simulink model "MassSpringDamper"  (R2021a)
settings: Solver=FixedStepAuto  StartTime=0.0  StopTime=10.0  FixedStep=0.01  RelTol=1e-3
model workspace (MAT data in the model file):
  b = 1
  k = 1
  m = 1
libraries: fl_lib x9, nesl_utility x6, sm_lib x4, fl_ps_legacy_lib x1
settings Model: Creator=yleong  LastModifiedBy=smuckati
settings SolverCC: AlgebraicLoopSolver=TrustRegion
settings OptimizationCC: DefaultParameterBehavior=Inlined  UseDivisionForNetSlopeComputation=on  EnhancedBackFolding=on  PassReuseOutputArgsAs=Individual arguments  OptimizeBlockOrder=speed  DifferentSizesBufferReuse=on  OptimizationCustomize=off  EfficientTunableParamExpr=on
settings DebuggingCC: ParameterTunabilityLossMsg=error  SFMachineParentedDataDiag=warning  ArithmeticOperatorsInVariantConditions=warning
settings SFSimCC: MATLABDynamicMemAlloc=off  CustomCodeUndefinedFunction=UseInterfaceOnly
settings RTWCC: SystemTargetFile=ert.tlc  TemplateMakefile=ert_default_tmf  IncludeHyperlinkInReport=on  CodeExecutionProfiling=on  CodeProfilingSaveOptions=AllData
settings CodeAppCC: ForceParamTrailComments=on  IgnoreCustomStorageClasses=off  OperatorAnnotations=on  SimulinkDataObjDesc=on  SFDataObjDesc=on  InsertBlockDesc=on
settings ERTTargetCC: TargetLangStandard=C99 (ISO)  GenerateSampleERTMain=on  InlinedParameterPlacement=NonHierarchical  ERTCustomFileTemplate=example_file_process.tlc

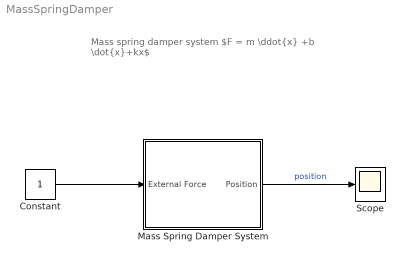
== system MassSpringDamper ==
  note: Mass spring damper system
      |
      | $F = m \ddot{x} +b \dot{x}+kx$
  " Scope " : Scope
  Constant : Constant
  Mass Spring Damper System : Subsystem  Variant=on  VariantControlMode=label  LabelModeActiveChoice=Equation of motion
  wires:
  Mass Spring Damper System/1(Position) -> " Scope "/1  "position"
  Constant/1 -> Mass Spring Damper System/1(" External Force")

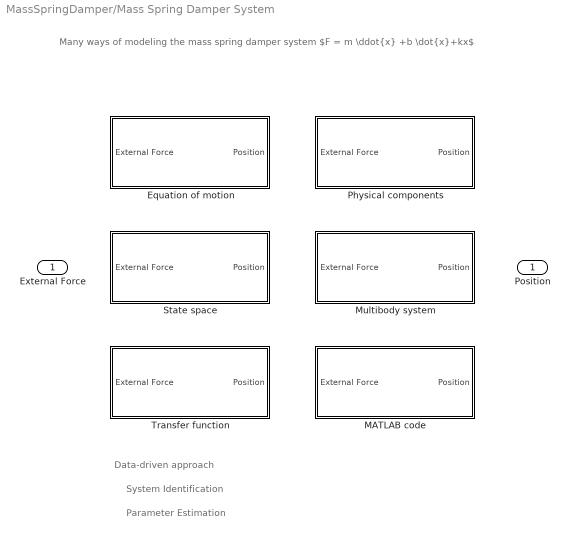
== system MassSpringDamper/Mass Spring Damper System ==
  note: Parameter Estimation
  note: Data-driven approach
  note: System Identification
  note: Many ways of modeling the mass spring damper system
      |
      | $F = m \ddot{x} +b \dot{x}+kx$
  " External Force" : Inport
  Equation of motion : Subsystem  VariantControl=Equation of motion
  MATLAB code : Subsystem  VariantControl=MATLAB code
  Multibody system : Subsystem  VariantControl=Multibody system
  Physical components : Subsystem  VariantControl=Physical components
  State space : Subsystem  VariantControl=State space
  Transfer function : Subsystem  VariantControl=Transfer function
  Position : Outport  VectorParamsAs1DForOutWhenUnconnected=off

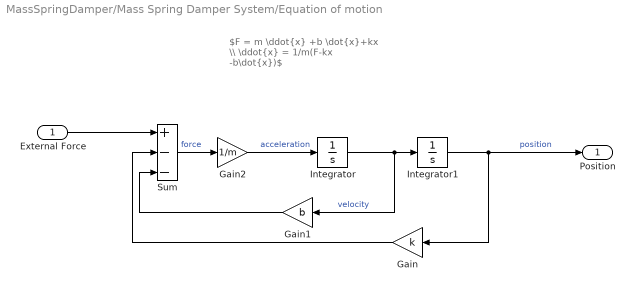
== system MassSpringDamper/Mass Spring Damper System/Equation of motion ==
  note: $F = m \ddot{x} +b \dot{x}+kx \\ \ddot{x} = 1/m(F-kx -b\dot{x})$
  " External Force" : Inport
  Gain : Gain  Gain=k
  Gain1 : Gain  Gain=b
  Gain2 : Gain  Gain=1/m
  Integrator : Integrator
  Integrator1 : Integrator
  Sum : Sum  Inputs=+--
  Position : Outport  VectorParamsAs1DForOutWhenUnconnected=off
  wires:
  Sum/1 -> Gain2/1  "force"
  Integrator1/1 -> Position/1, Gain/1  "position"
  Gain1/1 -> Sum/3
  Integrator/1 -> Gain1/1, Integrator1/1  "velocity"
  Gain/1 -> Sum/2
  Gain2/1 -> Integrator/1  "acceleration"
  " External Force"/1 -> Sum/1

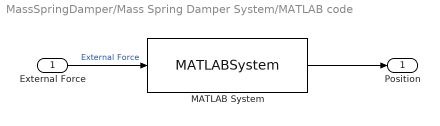
== system MassSpringDamper/Mass Spring Damper System/MATLAB code ==
  " External Force" : Inport
  MATLAB System : MATLABSystem  System=MassSpringDamperSystem  m=1  k=0.1  b=0.1  SimulateUsing=Code generation
      mask Type: MassSpringDamperSystem
      mask Display:
      | disp('MassSpringDamperSystem');
      | port_label('input',1,'u');
      | port_label('output',1,'y');
  Position : Outport  VectorParamsAs1DForOutWhenUnconnected=off
  wires:
  " External Force"/1 -> MATLAB System/1  "External Force"
  MATLAB System/1 -> Position/1

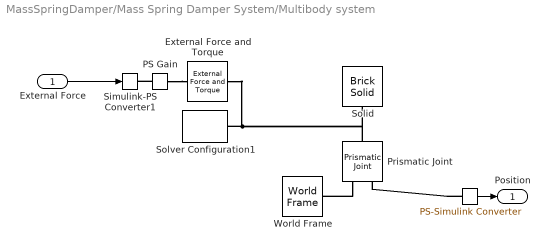
== system MassSpringDamper/Mass Spring Damper System/Multibody system ==
  " External Force" : Inport
  " " : nesl_utility/PS-Simulink Converter  PhysicalDomain=network_engine_domain  SubClassName=ps_output  LeftPortType=input  RightPortType=output  PseudoPeriodic=off  Frequencies=[]  Unit=1  AffineConversion=off
      settings: SourceProductBaseCode=PW,SS
  External Force and Torque : sm_lib/Forces and Torques/External Force and Torque  ForceResolutionFrame=AttachedFrame  EnableForceX=off  EnableForceY=off  EnableForceZ=on  EnableForce=off  TorqueResolutionFrame=AttachedFrame  EnableTorqueX=off  EnableTorqueY=off  EnableTorqueZ=off  EnableTorque=off
  PS Gain : fl_ps_legacy_lib/Legacy Physical Signals/Functions/PS Gain  gain=-1
  Prismatic Joint : sm_lib/Joints/Prismatic Joint  JointMode=Normal  SenseConstraintForce=off  SenseConstraintForceX=off  SenseConstraintForceY=off  SenseConstraintForceZ=off  SenseConstraintTorque=off  SenseConstraintTorqueX=off  SenseConstraintTorqueY=off  SenseConstraintTorqueZ=off  SenseTotalForce=off  SenseTotalForceX=off  SenseTotalForceY=off  SenseTotalForceZ=off  SenseTotalTorque=off  SenseTotalTorqueX=off  SenseTotalTorqueY=off  SenseTotalTorqueZ=off  CompositeWrenchDir=FollowerOnBase  CompositeWrenchFrame=BaseFrame  EquilibriumPosition=0  EquilibriumPositionUnits=m  SpringStiffness=k  SpringStiffnessUnits=N/m  DampingCoefficient=b  DampingCoefficientUnits=N/(m/s)  TorqueActuationMode=NoTorque  MotionActuationMode=ComputedMotion  SensePosition=on  SenseVelocity=off  SenseAcceleration=off  SenseTorqueForce=off  SenseLowerLimitTorqueForce=off  SenseUpperLimitTorqueForce=off  LowerLimitSpecify=off  LowerLimitBound=-1  LowerLimitBoundUnits=m  LowerLimitStiffness=1e6  LowerLimitStiffnessUnits=N/m  LowerLimitDamping=1e3  LowerLimitDampingUnits=N/(m/s)  LowerLimitTransitionRegionWidth=1e-4  LowerLimitTransitionRegionWidthUnits=m  UpperLimitSpecify=off  UpperLimitBound=1  UpperLimitBoundUnits=m  UpperLimitStiffness=1e6  UpperLimitStiffnessUnits=N/m  UpperLimitDamping=1e3  UpperLimitDampingUnits=N/(m/s)  UpperLimitTransitionRegionWidth=1e-4  UpperLimitTransitionRegionWidthUnits=m  PositionTargetSpecify=off  PositionTargetPriority=High  PositionTargetValue=10  PositionTargetValueUnits=m  VelocityTargetSpecify=off  VelocityTargetPriority=High  VelocityTargetValue=0  VelocityTargetValueUnits=m/s
  Simulink-PS Converter1 : nesl_utility/Simulink-PS Converter  PhysicalDomain=network_engine_domain  SubClassName=ps_input  LeftPortType=input  RightPortType=output  PseudoPeriodic=off  Frequencies=[]  NoiseDistribution=none  NoiseParameters=[]  Unit=N  AffineConversion=off  FilteringAndDerivatives=provide  SimscapeFilterOrder=1  InputFilterTimeConstant=0.001  UdotUserProvided=0
      settings: SourceProductBaseCode=PW,SS
  Solid : sm_lib/Body Elements/Brick Solid  GraphicAmbientColor=[0.15 0.15 0.15 1.0]  BasedOnType=Mass  BrickDimensions=[1 1 1]  BrickDimensionUnits=m  CenterOfMass=[0 0 0]  CenterOfMassUnits=m  GraphicDiffuseColor=[0.5 0.5 0.5]  Density=1000  DensityUnits=kg/m^3  DoExposeReferenceFrame=on  GraphicEmissiveColor=[0.0 0.0 0.0 1.0]  ExportEntireGeometry=off  SerializedFrames=<Frames/>  MarkerShape=Sphere  MarkerSize=10  GraphicType=FromGeometry  InertiaType=CalculateFromGeometry  Mass=m  MassUnits=kg  MomentsOfInertia=[1 1 1]  MomentsOfInertiaUnits=kg*m^2  GraphicOpacity=1.0  ProductsOfInertia=[0 0 0]  ProductsOfInertiaUnits=kg*m^2  GraphicShininess=75  GraphicSpecularColor=[0.5 0.5 0.5 1.0]  GraphicVisPropType=SimpleVisualProperties
  Solver Configuration1 : nesl_utility/Solver Configuration  PhysicalDomain=network_engine_domain  SubClassName=solver  LeftPortType=input  RightPortType=generic  Tones=[]  Harmonics=[]  SimulateNoise=off  Profile=off  UseLocalSampling=off  EnableSwitchedLinearOptims=on  FrequencyDomain=off  UseCCode=off  RelTol=0.001  AbsTol=1e-06  MinStep=1e-09  ToWorkspace=off  RevertToSquareIcSolve=off  NumHomotopyIterations=100  PhasorMode=off  PhasorModeNumHarmonics=1  DoDC=off  ResidualTolerance=1e-09  UseLocalSolver=off  LocalSolverChoice=NE_BACKWARD_EULER_ADVANCER  LocalSolverSampleTime=0.001  DoFixedCost=off  MaxNonlinIter=3  MaxModeIter=2  ComputeImpulses=off  ImpulseIterations=2  LinearAlgebra=auto  EquationFormulation=NE_TIME_EF  DelaysMemoryBudget=1024  AutomaticFiltering=on  FilteringTimeConstant=0.001  PartitionStorageMethod=AS_NEEDED  PartitionMemoryBudget=1024  PartitionMethod=FAST
      settings: SourceProductBaseCode=PW,SS
  World Frame : sm_lib/Frames and Transforms/World Frame
  Position : Outport  VectorParamsAs1DForOutWhenUnconnected=off
  wires:
  " External Force"/1 -> Simulink-PS Converter1/1
  " "/1 -> Position/1
  connections:
  Solver Configuration1/RConn1 -- Prismatic Joint/LConn1 -- Solid/RConn1 -- External Force and Torque/RConn1
  " "/LConn1 -- Prismatic Joint/RConn2
  Prismatic Joint/RConn1 -- World Frame/RConn1
  PS Gain/LConn1 -- Simulink-PS Converter1/RConn1
  PS Gain/RConn1 -- External Force and Torque/LConn1

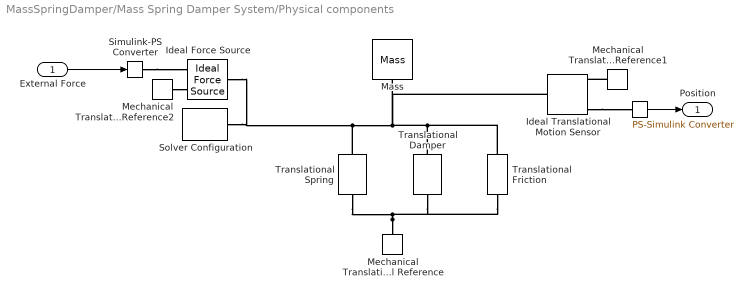
== system MassSpringDamper/Mass Spring Damper System/Physical components ==
  " External Force" : Inport
  " " : nesl_utility/PS-Simulink Converter  PhysicalDomain=network_engine_domain  SubClassName=ps_output  LeftPortType=input  RightPortType=output  PseudoPeriodic=off  Frequencies=[]  Unit=1  AffineConversion=off
      settings: SourceProductBaseCode=PW,SS
  Ideal Force Source : fl_lib/Mechanical/Mechanical Sources/Ideal Force Source
  Ideal Translational Motion Sensor : fl_lib/Mechanical/Mechanical Sensors/Ideal Translational Motion Sensor  offset=0 m
  Mass : fl_lib/Mechanical/Translational Elements/Mass  mass=m kg  num_ports=foundation.enum.numPorts2.one  v_specify=off  v_priority=High  v=0 m/s  v_nominal_specify=off  v_nominal_unit=m/s  v_nominal_value=1  f_specify=off  f_priority=None  f=0 N  f_nominal_specify=off  f_nominal_unit=N  f_nominal_value=1
  Mechanical Translational Reference : fl_lib/Mechanical/Translational Elements/Mechanical Translational Reference
  Mechanical Translational Reference1 : fl_lib/Mechanical/Translational Elements/Mechanical Translational Reference
  Mechanical Translational Reference2 : fl_lib/Mechanical/Translational Elements/Mechanical Translational Reference
  Simulink-PS Converter : nesl_utility/Simulink-PS Converter  PhysicalDomain=network_engine_domain  SubClassName=ps_input  LeftPortType=input  RightPortType=output  PseudoPeriodic=off  Frequencies=[]  NoiseDistribution=none  NoiseParameters=[]  Unit=N  AffineConversion=off  FilteringAndDerivatives=provide  SimscapeFilterOrder=1  InputFilterTimeConstant=0.001  UdotUserProvided=0
      settings: SourceProductBaseCode=PW,SS
  Solver Configuration : nesl_utility/Solver Configuration  PhysicalDomain=network_engine_domain  SubClassName=solver  LeftPortType=input  RightPortType=generic  Tones=[]  Harmonics=[]  SimulateNoise=off  Profile=off  UseLocalSampling=off  EnableSwitchedLinearOptims=on  FrequencyDomain=off  UseCCode=off  RelTol=0.001  AbsTol=1e-06  MinStep=1e-09  ToWorkspace=off  RevertToSquareIcSolve=off  NumHomotopyIterations=100  PhasorMode=off  PhasorModeNumHarmonics=1  DoDC=off  ResidualTolerance=1e-09  UseLocalSolver=off  LocalSolverChoice=NE_BACKWARD_EULER_ADVANCER  LocalSolverSampleTime=0.001  DoFixedCost=off  MaxNonlinIter=3  MaxModeIter=2  ComputeImpulses=off  ImpulseIterations=2  LinearAlgebra=auto  EquationFormulation=NE_TIME_EF  DelaysMemoryBudget=1024  AutomaticFiltering=on  FilteringTimeConstant=0.001  PartitionStorageMethod=AS_NEEDED  PartitionMemoryBudget=1024  PartitionMethod=FAST
      settings: SourceProductBaseCode=PW,SS
  Translational Friction : fl_lib/Mechanical/Translational Elements/Translational Friction  brkwy_frc=0.001 N  brkwy_vel=0.001 m/s  Col_frc=0.001 N  visc_coef=0.001 N/(m/s)  v_specify=off  v_priority=None  v=0 m/s  v_nominal_specify=off  v_nominal_unit=m/s  v_nominal_value=1  f_specify=off  f_priority=None  f=0 N  f_nominal_specify=off  f_nominal_unit=N  f_nominal_value=1
      settings: SourceProductBaseCode=SS  InternalSimscapePortConfiguration="{\"Bottom\":[],\"Left\":[{\"id\":\"R\",\"label\":\"R\",\"type\":\"foundation.mechanical.translational.translational\"}],\"Right\":[{\"id\":\"C\",\"label\":\"C\",\"type\":\"foundation.mechanical.translational.translational\"}],\"Top\":[]}"
  Translational Damper : fl_lib/Mechanical/Translational Elements/Translational Damper  D=b N/(m/s)  v_specify=off  v_priority=None  v=0 m/s  v_nominal_specify=off  v_nominal_unit=m/s  v_nominal_value=1  f_specify=off  f_priority=None  f=0 N  f_nominal_specify=off  f_nominal_unit=N  f_nominal_value=1
  Translational Spring : fl_lib/Mechanical/Translational Elements/Translational Spring  spr_rate=k N/m  v_specify=off  v_priority=None  v=0 m/s  v_nominal_specify=off  v_nominal_unit=m/s  v_nominal_value=1  f_specify=off  f_priority=None  f=0 N  f_nominal_specify=off  f_nominal_unit=N  f_nominal_value=1  x_specify=on  x_priority=None  x=0 m  x_nominal_specify=off  x_nominal_unit=m  x_nominal_value=1
  Position : Outport  VectorParamsAs1DForOutWhenUnconnected=off
  wires:
  " "/1 -> Position/1
  " External Force"/1 -> Simulink-PS Converter/1
  connections:
  Translational Damper/LConn1 -- Translational Spring/LConn1 -- Ideal Force Source/LConn1 -- Solver Configuration/RConn1 -- Ideal Translational Motion Sensor/LConn1 -- Mass/LConn1 -- Translational Friction/LConn1
  Mechanical Translational Reference/LConn1 -- Translational Friction/RConn1 -- Translational Damper/RConn1 -- Translational Spring/RConn1
  Mechanical Translational Reference2/LConn1 -- Ideal Force Source/RConn2
  Mechanical Translational Reference1/LConn1 -- Ideal Translational Motion Sensor/RConn1
  Simulink-PS Converter/RConn1 -- Ideal Force Source/RConn1
  Ideal Translational Motion Sensor/RConn3 -- " "/LConn1

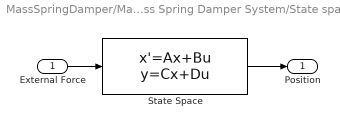
== system MassSpringDamper/Mass Spring Damper System/State space ==
  " External Force" : Inport
  State Space : StateSpace  A=[0 1; -k/m -b/m]  B=[0; 1/m]  C=[1 0]  D=0  InitialCondition=0
  Position : Outport  VectorParamsAs1DForOutWhenUnconnected=off
  wires:
  " External Force"/1 -> State Space/1
  State Space/1 -> Position/1

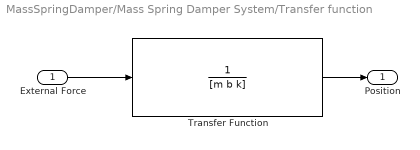
== system MassSpringDamper/Mass Spring Damper System/Transfer function ==
  " External Force" : Inport
  Transfer Function : TransferFcn  Denominator=[m b k]
  Position : Outport  VectorParamsAs1DForOutWhenUnconnected=off
  wires:
  Transfer Function/1 -> Position/1
  " External Force"/1 -> Transfer Function/1
